simulink model "sim"  (R2024a)
settings: Solver=FixedStepAuto  StartTime=0.0  StopTime=15.0  FixedStep=1e-3  RelTol=1e-3
settings Model: Creator=alexe  LastModifiedBy=alexe

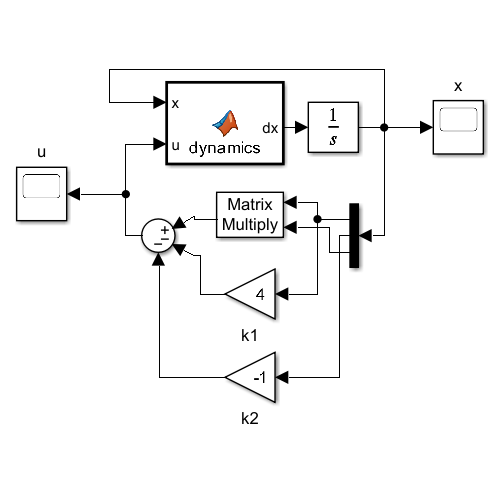
[thumbnail: Simulink's stored preview of the top-level diagram]
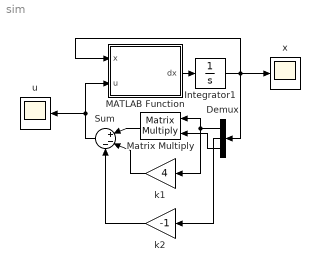
== system sim ==
  Demux : Demux  Outputs=3
  Integrator1 : Integrator  InitialCondition=[100; -70; 45];
  MATLAB Function : MATLAB Function  TreatAsAtomicUnit=on
  Matrix Multiply : Product  Multiplication=Matrix(*)
  Sum : Sum  Inputs=|+--
  k1 : Gain  Gain=4
  k2 : Gain  Gain=-1
  u : Scope
  x : Scope
  wires:
  Sum/1 -> u/1, MATLAB Function/2(u)
  MATLAB Function/1(dx) -> Integrator1/1
  Integrator1/1 -> Demux/1, MATLAB Function/1(x), x/1
  Demux/1 -> k1/1, Matrix Multiply/1
  Demux/3 -> Matrix Multiply/2
  Demux/2 -> k2/1
  Matrix Multiply/1 -> Sum/1
  k1/1 -> Sum/2
  k2/1 -> Sum/3

== matlab function sim/MATLAB Function ==
  data: x input; u input; dx output
function dx = dynamics(x, u)
    x1 = x(1);
    x2 = x(2);
    x3 = x(3);

    dx = zeros(3,1);
    dx(1) = -x1+x2;
    dx(2) = x1-x2-x1*x3+u;
    dx(3) = x1+x1*x2-2*x3;
end
